simulink model "buckboost_2016a"  (Simulink 8.7)
settings: Solver=ode23t  StartTime=0.0  StopTime=0.01  MaxStep=1e-7  RelTol=1e-3
libraries: powerlib x17, powerlib_meascontrol x3
settings Model: Creator=Asesh Kumar Seth  LastModifiedBy=sayan
settings DataIOCC: LimitDataPoints=off  SaveFormat=Dataset
settings DebuggingCC: UnderspecifiedInitializationDetection=Simplified  MergeDetectMultiDrivingBlocksExec=error
settings HardwareCC: ProdBitPerPointer=64  ProdLargestAtomicFloat=Float  ProdIntDivRoundTo=Zero  ProdEndianess=LittleEndian  ProdWordSize=64  ProdHWDeviceType=Intel->x86-64 (Windows64)
settings ModelReferenceCC: PropagateSignalLabelsOutOfModel=on
settings GRTTargetCC: GeneratePreprocessorConditionals=Use local settings
settings ConfigComp: CovModelRefEnable=off
settings SimscapeCC: SimscapeNormalizeSystem=off

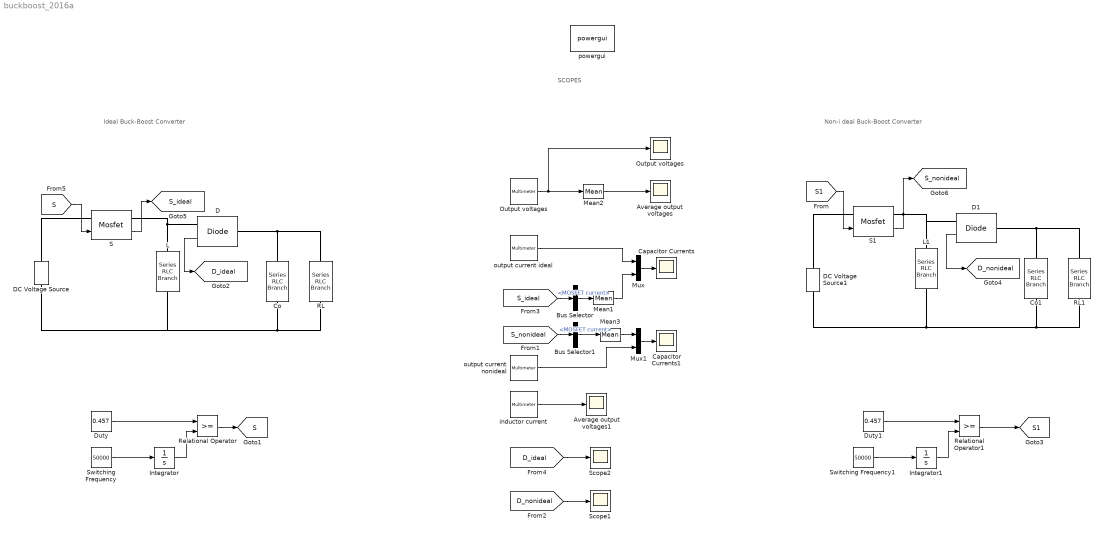
== system buckboost_2016a ==
  note: SCOPES
  note: Ideal Buck-Boost Converter
  note: Non-i deal Buck-Boost Converter
  Average output voltages : Scope
  Average output voltages1 : Scope
  Bus Selector : BusSelector  OutputSignals=MOSFET current
  Bus Selector1 : BusSelector  OutputSignals=MOSFET current
  Capacitor Currents : Scope
  Capacitor Currents1 : Scope
  Co : powerlib/Elements/Series RLC Branch  LConnTagsString=__new0  RConnTagsString=__new0  BranchType=C  Resistance=1  Inductance=1e-3  SetiL0=off  InitialCurrent=0  Capacitance=54e-6  Setx0=off  InitialVoltage=0  Measurements=Branch voltage and current
  Co1 : powerlib/Elements/Series RLC Branch  LConnTagsString=__new0  RConnTagsString=__new0  BranchType=C  Resistance=10e-3  Inductance=1e-3  SetiL0=off  InitialCurrent=0  Capacitance=54e-6  Setx0=off  InitialVoltage=0  Measurements=Branch voltage and current
  D : powerlib/Power Electronics/Diode  Ron=1e-6  Lon=0  Vf=0  IC=0  UseSnubber=off  Rs=1e5  Cs=inf  Measurements=on
  D1 : powerlib/Power Electronics/Diode  Ron=10e-3  Lon=0  Vf=0.7  IC=0  UseSnubber=off  Rs=1e5  Cs=inf  Measurements=on
  DC Voltage Source : powerlib/Electrical Sources/DC Voltage Source  Amplitude=57  Measurements=None
  DC Voltage Source1 : powerlib/Electrical Sources/DC Voltage Source  Amplitude=57  Measurements=None
  Duty : Constant  Value=0.457
  Duty1 : Constant  Value=0.457
  Integrator : Integrator  UpperSaturationLimit=1  LowerSaturationLimit=0  WrapState=on  WrappedStateUpperValue=1  WrappedStateLowerValue=0
  Integrator1 : Integrator  UpperSaturationLimit=1  LowerSaturationLimit=0  WrapState=on  WrappedStateUpperValue=1  WrappedStateLowerValue=0
  L : powerlib/Elements/Series RLC Branch  LConnTagsString=__new0  RConnTagsString=__new0  BranchType=L  Resistance=11.52*0.05  Inductance=226e-6  SetiL0=off  InitialCurrent=0  Capacitance=1e-6  Setx0=off  InitialVoltage=0  Measurements=Branch voltage and current
  L1 : powerlib/Elements/Series RLC Branch  LConnTagsString=__new0  RConnTagsString=__new0  BranchType=RL  Resistance=0.576  Inductance=226e-6  SetiL0=off  InitialCurrent=0  Capacitance=1e-6  Setx0=off  InitialVoltage=0  Measurements=Branch voltage and current
  Mean1 : powerlib_meascontrol/Measurements/Mean  Freq=50e3  Vinit=0  Ts=0
  Mean2 : powerlib_meascontrol/Measurements/Mean  Freq=50e3  Vinit=0  Ts=0
  Mean3 : powerlib_meascontrol/Measurements/Mean  Freq=50e3  Vinit=0  Ts=0
  Mux : Mux  Inputs=2
  Mux1 : Mux  Inputs=2
  Output voltages : Scope
  "Output voltages  " : powerlib/Measurements/Multimeter  PhasorSimulation=off  OutputType=Complex  sel=[5 6]  L=12  Gain=[1 1]  yselected={'Ub: RL','Ub: RL1'};  PSBOutputType=1  PSBequivalent=0  AxesSetting=[0,0.1,-100,100]  Display=0  SavedBlockNames=-11
  RL : powerlib/Elements/Series RLC Branch  LConnTagsString=__new0  RConnTagsString=__new0  BranchType=R  Resistance=11.52  Inductance=1e-3  SetiL0=off  InitialCurrent=0  Capacitance=1e-6  Setx0=off  InitialVoltage=0  Measurements=Branch voltage and current
  RL1 : powerlib/Elements/Series RLC Branch  LConnTagsString=__new0  RConnTagsString=__new0  BranchType=R  Resistance=11.52  Inductance=1e-3  SetiL0=off  InitialCurrent=0  Capacitance=1e-6  Setx0=off  InitialVoltage=0  Measurements=Branch voltage and current
  Relational Operator : RelationalOperator  OutDataTypeStr=boolean
  Relational Operator1 : RelationalOperator  OutDataTypeStr=boolean
  S : powerlib/Power Electronics/Mosfet  Ron=1e-6  Lon=1e-10  Rd=1e-10  Vfd=0  IC=0  Rs=1e5  Cs=inf  Measurements=on
  S1 : powerlib/Power Electronics/Mosfet  Ron=50e-3  Lon=1e-10  Rd=1e-10  Vfd=0  IC=0  Rs=1e5  Cs=inf  Measurements=on
  Scope1 : Scope
  Scope2 : Scope
  Switching Frequency : Constant  Value=50000
  Switching Frequency1 : Constant  Value=50000
  inductor current : powerlib/Measurements/Multimeter  PhasorSimulation=off  OutputType=Complex  sel=[9 10]  L=12  Gain=[1 1]  yselected={'Ib: L','Ib: L1'};  PSBOutputType=1  PSBequivalent=0  AxesSetting=[0,0.1,-100,100]  Display=0  SavedBlockNames=-11
  output current ideal : powerlib/Measurements/Multimeter  PhasorSimulation=off  OutputType=Complex  sel=11  L=12  Gain=1  yselected={'Ib: RL'};  PSBOutputType=1  PSBequivalent=0  AxesSetting=[0,0.1,-100,100]  Display=0  SavedBlockNames=-11
  output current nonideal : powerlib/Measurements/Multimeter  PhasorSimulation=off  OutputType=Complex  sel=12  L=12  Gain=1  yselected={'Ib: RL1'};  PSBOutputType=1  PSBequivalent=0  AxesSetting=[0,0.1,-100,100]  Display=0  SavedBlockNames=-11
  powergui : powerlib/powergui  Priority=1  SimulationMode=Discrete  SampleTime=5e-8  frequency=60  Iterations=50  frequencyindice=0  Pbase=100e6  ErrMax=1e-4  UnitsV=kV  UnitsW=MW  buscounter=0  FunctionMessages=off  echomessages=off  EnableUseOfTLC=off  CurrentSourceSwitches=on  DisableSnubberDevices=off  DisableRonSwitches=off  DisableVfSwitches=off  DisplayEquations=off  SolverType=Tustin/Backward Euler (TBE)  Interpol=off  ExternalGateDelay=off  methode=off  Ts=10  x0status=blocks  SPID=off  SwTol=0  HookPort=off  RestoreLinks=warning  ResistiveCurrentMeasurement=off  Frange=[0:2:500]  Ylog=off  Xlog=on  ShowGrid=off  save=off  variable=ZData  structure=0  ZoomFFT=off  StartTime=0.0  cycles=1  DisplayStyle=1  fundamental=60  FreqAxis=off  MaxFrequency=1000  frequencyindicesteady=1  RmsSteady=1  display=off
  tag scope: D_ideal=global, D_nonideal=global, S1=global, S=global, S_ideal=global, S_nonideal=global
  wires:
  Switching Frequency/1 -> Integrator/1
  Integrator/1 -> Relational Operator/2
  Duty/1 -> Relational Operator/1
  Mux/1 -> Capacitor Currents/1
  [D_ideal] -> Scope2/1
  D/1 -> [D_ideal]
  D1/1 -> [D_nonideal]
  Duty1/1 -> Relational Operator1/1
  Switching Frequency1/1 -> Integrator1/1
  Integrator1/1 -> Relational Operator1/2
  Relational Operator1/1 -> [S1]
  [S_nonideal] -> Bus Selector1/1
  [S_ideal] -> Bus Selector/1
  [D_nonideal] -> Scope1/1
  "Output voltages  "/1 -> Output voltages/1, Mean2/1
  Mean2/1 -> Average output voltages/1
  Relational Operator/1 -> [S]
  [S1] -> S1/1
  [S] -> S/1
  S/1 -> [S_ideal]
  S1/1 -> [S_nonideal]
  Bus Selector/1 -> Mean1/1  "<MOSFET current>"
  output current ideal/1 -> Mux/1
  Mean1/1 -> Mux/2
  Bus Selector1/1 -> Mean3/1  "<MOSFET current>"
  Mean3/1 -> Mux1/1
  output current nonideal/1 -> Mux1/2
  Mux1/1 -> Capacitor Currents1/1
  inductor current/1 -> Average output voltages1/1
  connections:
  D/LConn1 -- RL/RConn1 -- Co/RConn1
  Co/LConn1 -- RL/LConn1 -- L/RConn1 -- DC Voltage Source/LConn1
  DC Voltage Source/RConn1 -- S/LConn1
  L/LConn1 -- D/RConn1 -- S/RConn1
  S1/RConn1 -- L1/LConn1 -- D1/RConn1
  D1/LConn1 -- RL1/RConn1 -- Co1/RConn1
  L1/RConn1 -- DC Voltage Source1/LConn1 -- RL1/LConn1 -- Co1/LConn1
  DC Voltage Source1/RConn1 -- S1/LConn1
